simulink model "W"  (R2019b)
settings: Solver=VariableStepAuto  StartTime=0.0  StopTime=10.0  RelTol=1e-3
settings Model: Creator=enrique.babio  LastModifiedBy=enrique.babio
settings DataIOCC: SaveOutput=off  SaveTime=off

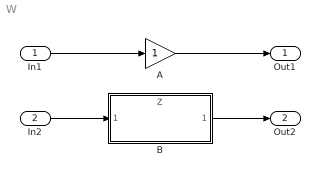
== system W ==
  In1 : Inport  OutDataTypeStr=double  PortDimensions=1
  In2 : Inport  Port=2  OutDataTypeStr=double  PortDimensions=1
  A : Gain
  B : ModelReference  ModelNameDialog=Z  SimulationMode=Normal  ModelReferenceVersion=1.3
  Out1 : Outport  OutDataTypeStr=double  PortDimensions=1
  Out2 : Outport  Port=2  OutDataTypeStr=double  PortDimensions=1
  wires:
  In1/1 -> A/1
  A/1 -> Out1/1
  In2/1 -> B/1
  B/1 -> Out2/1
